simulink model "fault_validation"  (R2021a)
settings: Solver=VariableStepAuto  StartTime=0.0  StopTime=1.0  RelTol=1e-3
undefined symbols (not defined in the file): D1, Delta
libraries: spsThreePhasePISectionLineLib x3, spsThreePhaseTransformerTwoWindingsLib x2, spsThreePhaseSourceLib x2, spsThreePhaseFaultLib x1, spsThreePhaseVIMeasurementLib x1, spspowerguiLib x1
settings Model: Creator=Prakhar  LastModifiedBy=Prakhar

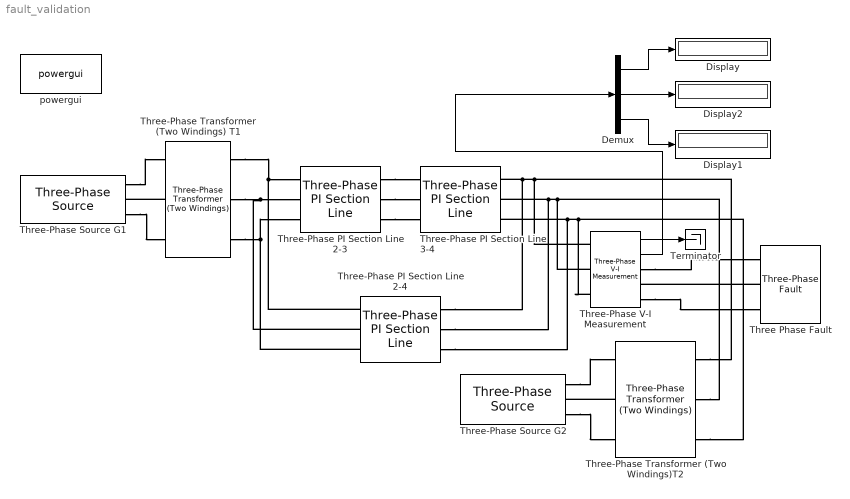
== system fault_validation ==
  Demux : Demux  Outputs=3
  Display : Display
  Display1 : Display
  Display2 : Display
  Terminator : Terminator
  Three Phase Fault : spsThreePhaseFaultLib/Three-Phase Fault  InitialStates=1  FaultA=off  FaultB=on  FaultC=on  GroundFault=on  SwitchTimes="[100  101]"  External=off  SwitchStatus=NaN  FaultResistance=1e-3  GroundResistance=1e-3  SnubberResistance=1e6  SnubberCapacitance=inf  Measurements=None
  Three-Phase PI Section Line 2-3 : spsThreePhasePISectionLineLib/Three-Phase PI Section Line  LConnTagsString=a|b|c  RConnTagsString=A|B|C  Length=1  Frequency=60  Resistances=[ 3.4848 10.4544]  Inductances="[ 0.046215  0.138645]"  Capacitances=[1e-7 1e-7]
  Three-Phase PI Section Line 2-4 : spsThreePhasePISectionLineLib/Three-Phase PI Section Line  LConnTagsString=a|b|c  RConnTagsString=A|B|C  Length=1  Frequency=60  Resistances=[ 5.2272 15.6816]  Inductances="[ 0.055444  0.166333]"  Capacitances=[1e-7 1e-7]
  Three-Phase PI Section Line 3-4 : spsThreePhasePISectionLineLib/Three-Phase PI Section Line  LConnTagsString=a|b|c  RConnTagsString=A|B|C  Length=1  Frequency=60  Resistances=[ 3.4848 10.4544]  Inductances="[ 0.036973  0.110918]"  Capacitances=[1e-7 1e-7]
  Three-Phase Transformer (Two Windings) T1 : spsThreePhaseTransformerTwoWindingsLib/Three-Phase Transformer (Two Windings)  Winding1Connection=Delta (D1)  Winding2Connection=Yg  CoreType=Three single-phase transformers  SetSaturation=off  Hysteresis=off  DataFile='hysteresis'  SetInitialFlux=off  Measurements=None  UNITS=pu  NominalPower=[ 100e6 , 60 ]  Winding1=[ 11e3 , 0 , 0.05 ]  Winding2=[ 132e3 , 0 , 0.05 ]  Rm=500  Lm=500  L0=0.5  Saturation=[ 0,0 ; 0.0024,1.2 ; 1.0,1.52 ]  InitialFluxes=[ 0.8 , -0.8 , 0.7 ]  BreakLoop=off  DiscreteSolver=Trapezoidal iterative  DataType=off  TransfoNumber=1
  Three-Phase Transformer (Two Windings)T2 : spsThreePhaseTransformerTwoWindingsLib/Three-Phase Transformer (Two Windings)  Winding1Connection=Delta (D1)  Winding2Connection=Yg  CoreType=Three single-phase transformers  SetSaturation=off  Hysteresis=off  DataFile='hysteresis'  SetInitialFlux=off  Measurements=None  UNITS=pu  NominalPower=[ 100e6 , 60 ]  Winding1=[ 11e3 , 0 , 0.06 ]  Winding2=[ 132e3 , 0 , 0.06 ]  Rm=500  Lm=500  L0=0.5  Saturation=[ 0,0 ; 0.0024,1.2 ; 1.0,1.52 ]  InitialFluxes=[ 0.8 , -0.8 , 0.7 ]  BreakLoop=off  DiscreteSolver=Trapezoidal iterative  DataType=off  TransfoNumber=1
  Three-Phase V-I Measurement : spsThreePhaseVIMeasurementLib/Three-Phase V-I Measurement  VoltageMeasurement=phase-to-ground  SetLabelV=off  LabelV=Vabc  Vpu=off  VpuLL=off  CurrentMeasurement=yes  SetLabelI=off  LabelI=Iabc  Ipu=off  Pbase=100e6  Vbase=500e3  OutputType=Complex  PhasorSimulation=on  PSBequivalent=0
  Three-Phase Source G1 : spsThreePhaseSourceLib/Three-Phase Source  InternalConnection=Yg  VoltagePhases=off  Voltage=11e3  PhaseAngle=0  Voltage_phases=[25e3 25e3 25e3]/sqrt(3)  PhaseAngles_phases=[0 -120 +120]  Frequency=60  NonIdealSource=on  SpecifyImpedance=off  Resistance=0  Inductance=4.816e-4  ShortCircuitLevel=100e6  BaseVoltage=11e3  XRratio=7  BusType=swing  Pref=10e3  Qref=0  Prefabc=[10e3, 10e3, 10e3]  Qrefabc=[0, 0, 0]  Qmin=-inf  Qmax=inf
  Three-Phase Source G2 : spsThreePhaseSourceLib/Three-Phase Source  InternalConnection=Yg  VoltagePhases=off  Voltage=11e3  PhaseAngle=0  Voltage_phases=[25e3 25e3 25e3]/sqrt(3)  PhaseAngles_phases=[0 -120 +120]  Frequency=60  NonIdealSource=on  SpecifyImpedance=off  Resistance=0  Inductance=6.411e-4  ShortCircuitLevel=100e6  BaseVoltage=11e3  XRratio=7  BusType=swing  Pref=10e3  Qref=0  Prefabc=[10e3, 10e3, 10e3]  Qrefabc=[0, 0, 0]  Qmin=-inf  Qmax=inf
  powergui : spspowerguiLib/powergui  Priority=1  SimulationMode=Phasor  SampleTime=50e-6  frequency=60  Iterations=50  frequencyindice=60  Pbase=100e6  ErrMax=1e-4  UnitsV=kV  UnitsW=MW  buscounter=0  FunctionMessages=off  echomessages=off  EnableUseOfTLC=off  CurrentSourceSwitches=off  DisableSnubberDevices=off  DisableRonSwitches=off  DisableVfSwitches=off  DisplayEquations=off  AutomaticDiscreteSolvers=off  SolverType=Tustin/Backward Euler (TBE)  Interpol=off  ExternalGateDelay=off  methode=off  Ts=100  x0status=blocks  SPID=on  SwTol=0  HookPort=off  NonlinearTolerance=1e-4  nMaxIteration=100  ContinueOnMaxIteration=off  RestoreLinks=warning  ResistiveCurrentMeasurement=off  Frange=[0:2:500]  Ylog=off  Xlog=on  ShowGrid=off  save=on  variable=ZData  structure=0  ZoomFFT=off  StartTime=0.0  cycles=1  DisplayStyle=1  fundamental=60  FreqAxis=off  MaxFrequency=1000  frequencyindicesteady=1  RmsSteady=1  display=off
  wires:
  Three-Phase V-I Measurement/2 -> Demux/1
  Three-Phase V-I Measurement/1 -> Terminator/1
  Demux/1 -> Display/1
  Demux/2 -> Display2/1
  Demux/3 -> Display1/1
  connections:
  Three-Phase Transformer (Two Windings) T1/LConn2 -- Three-Phase Source G1/RConn2
  Three-Phase Source G1/RConn1 -- Three-Phase Transformer (Two Windings) T1/LConn1
  Three-Phase Source G1/RConn3 -- Three-Phase Transformer (Two Windings) T1/LConn3
  Three-Phase Transformer (Two Windings) T1/RConn1 -- Three-Phase PI Section Line 2-4/LConn1 -- Three-Phase PI Section Line 2-3/LConn1
  Three-Phase Transformer (Two Windings) T1/RConn2 -- Three-Phase PI Section Line 2-4/LConn2 -- Three-Phase PI Section Line 2-3/LConn2
  Three-Phase Transformer (Two Windings) T1/RConn3 -- Three-Phase PI Section Line 2-3/LConn3 -- Three-Phase PI Section Line 2-4/LConn3
  Three-Phase PI Section Line 2-3/RConn1 -- Three-Phase PI Section Line 3-4/LConn1
  Three-Phase PI Section Line 2-3/RConn2 -- Three-Phase PI Section Line 3-4/LConn2
  Three-Phase PI Section Line 2-3/RConn3 -- Three-Phase PI Section Line 3-4/LConn3
  Three-Phase Transformer (Two Windings)T2/LConn2 -- Three-Phase Source G2/RConn2
  Three-Phase Source G2/RConn1 -- Three-Phase Transformer (Two Windings)T2/LConn1
  Three-Phase Source G2/RConn3 -- Three-Phase Transformer (Two Windings)T2/LConn3
  Three-Phase Transformer (Two Windings)T2/RConn1 -- Three-Phase V-I Measurement/LConn1 -- Three-Phase PI Section Line 2-4/RConn1 -- Three-Phase PI Section Line 3-4/RConn1
  Three-Phase Transformer (Two Windings)T2/RConn2 -- Three-Phase V-I Measurement/LConn2 -- Three-Phase PI Section Line 2-4/RConn2 -- Three-Phase PI Section Line 3-4/RConn2
  Three-Phase Transformer (Two Windings)T2/RConn3 -- Three-Phase V-I Measurement/LConn3 -- Three-Phase PI Section Line 2-4/RConn3 -- Three-Phase PI Section Line 3-4/RConn3
  Three Phase Fault/LConn2 -- Three-Phase V-I Measurement/RConn2
  Three-Phase V-I Measurement/RConn1 -- Three Phase Fault/LConn1
  Three-Phase V-I Measurement/RConn3 -- Three Phase Fault/LConn3
